simulink model "sldemo_hydcyl4"  (R2022b)
settings: Solver=ode45  StartTime=0.0  StopTime=0.1  FixedStep=0.001  RelTol=1e-6
model workspace (MATLAB code in the model file):
  | % Load the initial conditions and initialization data
  | % Using the same MAT file as
  | % sldemo_hydcyl
  | % sldemo_hydcyl4
  | % sldemo_hydrod
  | 
  | load sldemo_hydcyl_data;
undefined symbols (not defined in the file or in its folder): Ac, Beta, K, Qmax
libraries: hydlib x5
Description:
  | Four Hydraulic Cylinder Simulation
  | 
  | This example uses Simulink(R) to create a model with four hydraulic cylinders. See
  | two related examples that use the same basic components:
  | 
  | * single cylinder model: sldemo_hydcyl
  | * model with two cylinders and load constraints: sldemo_hydrod
settings Model: Creator=The MathWorks, Inc.  LastModifiedBy=The MathWorks, Inc.
settings SolverCC: AlgebraicLoopSolver=TrustRegion
settings DataIOCC: SaveFormat=Array  SaveOutput=off  SaveTime=off  SignalLoggingName=sldemo_hydcyl4_output
settings OptimizationCC: BooleanDataType=off  ExpressionDepthLimit=2147483647  InitFltsAndDblsToZero=on  LifeSpan=inf  BufferReusableBoundary=off
settings DebuggingCC: AlgebraicLoopMsg=none  SaveWithParameterizedLinksMsg=none  UnderspecifiedInitializationDetection=Classic  MergeDetectMultiDrivingBlocksExec=none  SignalResolutionControl=TryResolveAllWithWarning  MultiTaskDSMMsg=warning  MultiTaskCondExecSysMsg=none  SigSpecEnsureSampleTimeMsg=none  IntegerOverflowMsg=none  FcnCallInpInsideContextMsg=warning  UnconnectedInputMsg=warning  UnconnectedOutputMsg=warning  UnconnectedLineMsg=warning  BusObjectLabelMismatch=none  StateNameClashWarn=warning  SFUnexpectedBacktrackingDiag=warning  SFNoUnconditionalDefaultTransitionDiag=warning  SFExecutionAtInitializationDiag=none  SFMachineParentedDataDiag=warning  IntegerSaturationMsg=none  ArithmeticOperatorsInVariantConditions=warning
settings HardwareCC: ProdBitPerPointer=32  ProdBitPerSizeT=32  ProdBitPerPtrDiffT=32  ProdLargestAtomicFloat=None  ProdIntDivRoundTo=Undefined  ProdEndianess=Unspecified  ProdWordSize=32  ProdHWDeviceType=32-bit Generic  TargetUnknown=on
settings ModelReferenceCC: EnableRefExpFcnMdlSchedulingChecks=on  PropagateSignalLabelsOutOfModel=off
settings SFSimCC: SimUseLocalCustomCode=off  CustomCodeUndefinedFunction=UseInterfaceOnly
settings RTWCC: RTWUseLocalCustomCode=off
settings CodeAppCC: StateflowObjectComments=on
settings GRTTargetCC: TargetFcnLib=ansi_tfl_tmw.mat  TargetLangStandard=C89/C90 (ANSI)  CombineOutputUpdateFcns=off  GRTInterface=on
settings ConfigComp: CovMetricSettings=dw  CovSaveCumulativeToWorkspaceVar=on  CovSaveSingleToWorkspaceVar=on  CovExternalEMLEnable=off

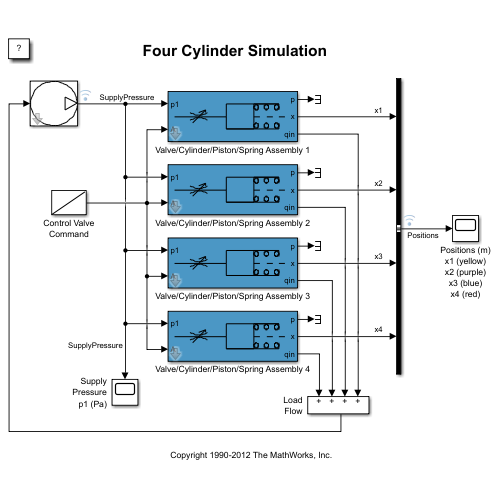
[thumbnail: Simulink's stored preview of the top-level diagram]
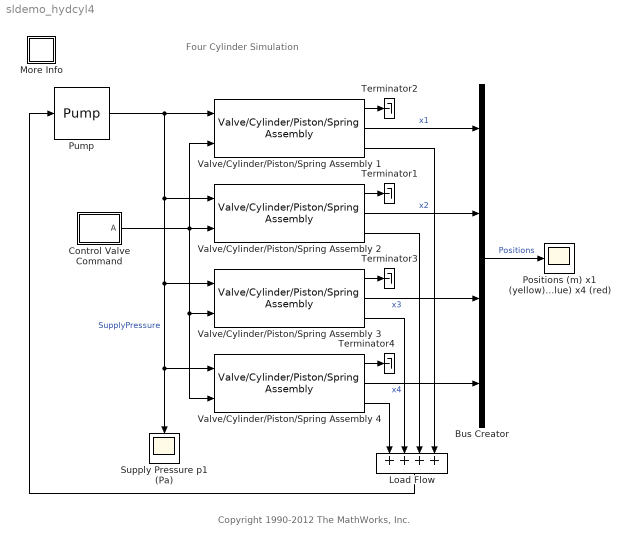
== system sldemo_hydcyl4 ==
  note: Four Cylinder Simulation
  note: Copyright 1990-2012 The MathWorks, Inc.
  Bus Creator : BusCreator  Inputs=4
  Control Valve Command : Subsystem  mask(Ramp){}
      mask Display: plot(0,0,100,100,[98,0],[96,0])
  Load Flow : Sum  Inputs=++++  InputSameDT=on  SaturateOnIntegerOverflow=on  OutDataTypeStr=Inherit: Same as first input
  More Info : Subsystem
      settings: OpenFcn=showExample('simulink_general/sldemo_hydcyl4Example')
      mask Display: disp('?')
  Positions (m) x1 (yellow) x2 (purple) x3 (blue) x4 (red) : Scope
  Pump : hydlib/Pump  t=[0 0.05 0.051 0.1]  Qpump=Qmax*[1 1 0.5 0.5]  p10=Qmax/C2/2  C2=C2
  Supply Pressure p1 (Pa) : Scope
  Terminator{1..4} (4 alike) : Terminator
  Valve/Cylinder/Piston/Spring Assembly 1 : hydlib/Valve//Cylinder//Piston//Spring Assembly  K=K  C1=C1  Ac=Ac  Cd=Cd  rho=rho  V30=V30  beta=Beta  assemblyName=Spring1
  Valve/Cylinder/Piston/Spring Assembly 2 : hydlib/Valve//Cylinder//Piston//Spring Assembly  K=K/4  C1=C1  Ac=Ac/4  Cd=Cd  rho=rho  V30=V30  beta=Beta  assemblyName=Spring2
  Valve/Cylinder/Piston/Spring Assembly 3 : hydlib/Valve//Cylinder//Piston//Spring Assembly  K=K*4  C1=C1  Ac=Ac*4  Cd=Cd  rho=rho  V30=V30  beta=Beta  assemblyName=Spring3
  Valve/Cylinder/Piston/Spring Assembly 4 : hydlib/Valve//Cylinder//Piston//Spring Assembly  K=K  C1=C1  Ac=Ac  Cd=Cd  rho=rho  V30=V30  beta=Beta/1000  assemblyName=Spring4
  wires:
  Valve/Cylinder/Piston/Spring Assembly 4/1 -> Terminator4/1
  Valve/Cylinder/Piston/Spring Assembly 3/1 -> Terminator3/1
  Valve/Cylinder/Piston/Spring Assembly 2/1 -> Terminator1/1
  Valve/Cylinder/Piston/Spring Assembly 1/1 -> Terminator2/1
  Load Flow/1 -> Pump/1
  Valve/Cylinder/Piston/Spring Assembly 1/3 -> Load Flow/4
  Valve/Cylinder/Piston/Spring Assembly 2/3 -> Load Flow/3
  Valve/Cylinder/Piston/Spring Assembly 3/3 -> Load Flow/2
  Valve/Cylinder/Piston/Spring Assembly 4/3 -> Load Flow/1
  Valve/Cylinder/Piston/Spring Assembly 2/2 -> Bus Creator/2  "x2"
  Valve/Cylinder/Piston/Spring Assembly 4/2 -> Bus Creator/4  "x4"
  Valve/Cylinder/Piston/Spring Assembly 3/2 -> Bus Creator/3  "x3"
  Valve/Cylinder/Piston/Spring Assembly 1/2 -> Bus Creator/1  "x1"
  Control Valve Command/1(A) -> Valve/Cylinder/Piston/Spring Assembly 3/2, Valve/Cylinder/Piston/Spring Assembly 4/2, Valve/Cylinder/Piston/Spring Assembly 2/2, Valve/Cylinder/Piston/Spring Assembly 1/2
  Pump/1 -> Valve/Cylinder/Piston/Spring Assembly 2/1, Supply Pressure p1 (Pa)/1, Valve/Cylinder/Piston/Spring Assembly 4/1, Valve/Cylinder/Piston/Spring Assembly 3/1, Valve/Cylinder/Piston/Spring Assembly 1/1  "SupplyPressure"
  Bus Creator/1 -> Positions (m) x1 (yellow) x2 (purple) x3 (blue) x4 (red)/1  "Positions"

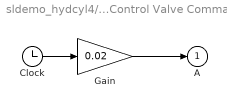
== system sldemo_hydcyl4/Control Valve Command ==
  Clock : Clock
  Gain : Gain  Gain=0.02  SaturateOnIntegerOverflow=on  OutDataTypeStr=Inherit: Same as input  ParamDataTypeStr=Inherit: Same as input
  A : Outport  InitialOutput=0  VectorParamsAs1DForOutWhenUnconnected=off
  wires:
  Clock/1 -> Gain/1
  Gain/1 -> A/1

== system sldemo_hydcyl4/More Info ==
